simulink model "Battery_Digital_Twin"  (R2026a)
settings: Solver=VariableStepAuto  StopTime=300
undefined symbols (not defined in the file): Battery, BMS, Sensors
libraries: simulink x6
settings Model: Creator=tastytaco  LastModifiedBy=tastytaco

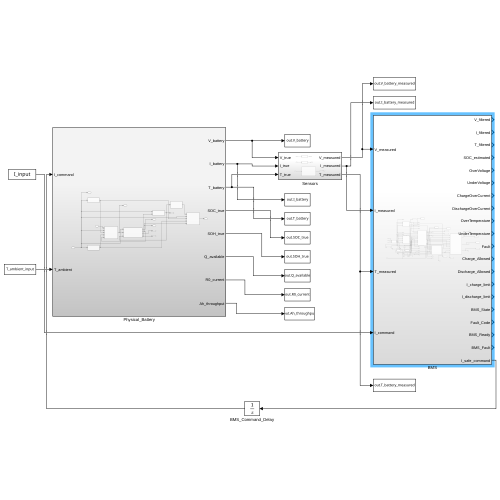
[thumbnail: Simulink's stored preview of the top-level diagram]
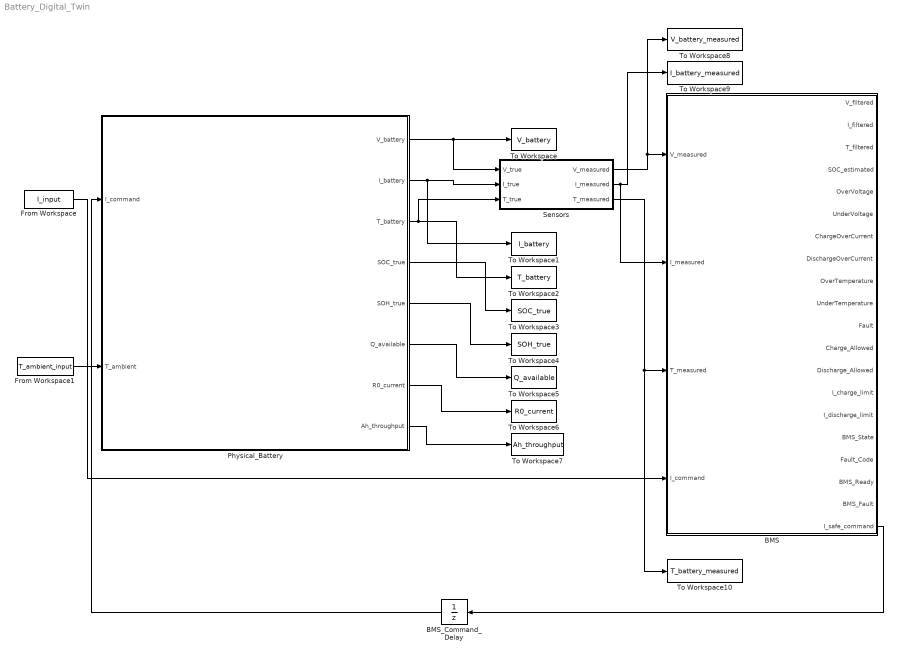
== system Battery_Digital_Twin ==
  BMS : Subsystem
  BMS_Command_Delay : UnitDelay  SampleTime=BMS.Ts
  From Workspace : FromWorkspace  VariableName=I_input
  From Workspace1 : FromWorkspace  VariableName=T_ambient_input
  Physical_Battery : Subsystem
  Sensors : Subsystem
  To Workspace : ToWorkspace  VariableName=V_battery  SaveFormat=Timeseries  SampleTime=-1
  To Workspace1 : ToWorkspace  VariableName=I_battery  SaveFormat=Timeseries  SampleTime=-1
  To Workspace10 : ToWorkspace  VariableName=T_battery_measured  SaveFormat=Timeseries  SampleTime=-1
  To Workspace2 : ToWorkspace  VariableName=T_battery  SaveFormat=Timeseries  SampleTime=-1
  To Workspace3 : ToWorkspace  VariableName=SOC_true  SaveFormat=Timeseries  SampleTime=-1
  To Workspace4 : ToWorkspace  VariableName=SOH_true  SaveFormat=Timeseries  SampleTime=-1
  To Workspace5 : ToWorkspace  VariableName=Q_available  SaveFormat=Timeseries  SampleTime=-1
  To Workspace6 : ToWorkspace  VariableName=R0_current  SaveFormat=Timeseries  SampleTime=-1
  To Workspace7 : ToWorkspace  VariableName=Ah_throughput  SaveFormat=Timeseries  SampleTime=-1
  To Workspace8 : ToWorkspace  VariableName=V_battery_measured  SaveFormat=Timeseries  SampleTime=-1
  To Workspace9 : ToWorkspace  VariableName=I_battery_measured  SaveFormat=Timeseries  SampleTime=-1
  wires:
  Sensors/3(T_measured) -> To Workspace10/1, BMS/3(T_measured)
  Physical_Battery/8(Ah_throughput) -> To Workspace7/1
  Physical_Battery/6(Q_available) -> To Workspace5/1
  Physical_Battery/5(SOH_true) -> To Workspace4/1
  Sensors/1(V_measured) -> BMS/1(V_measured), To Workspace8/1
  Physical_Battery/3(T_battery) -> To Workspace2/1, Sensors/3(T_true)
  Physical_Battery/1(V_battery) -> To Workspace/1, Sensors/1(V_true)
  Physical_Battery/2(I_battery) -> To Workspace1/1, Sensors/2(I_true)
  From Workspace1/1 -> Physical_Battery/2(T_ambient)
  Sensors/2(I_measured) -> BMS/2(I_measured), To Workspace9/1
  Physical_Battery/7(R0_current) -> To Workspace6/1
  Physical_Battery/4(SOC_true) -> To Workspace3/1
  From Workspace/1 -> BMS/4(I_command)
  BMS/20(I_safe_command) -> BMS_Command_Delay/1
  BMS_Command_Delay/1 -> Physical_Battery/1(I_command)

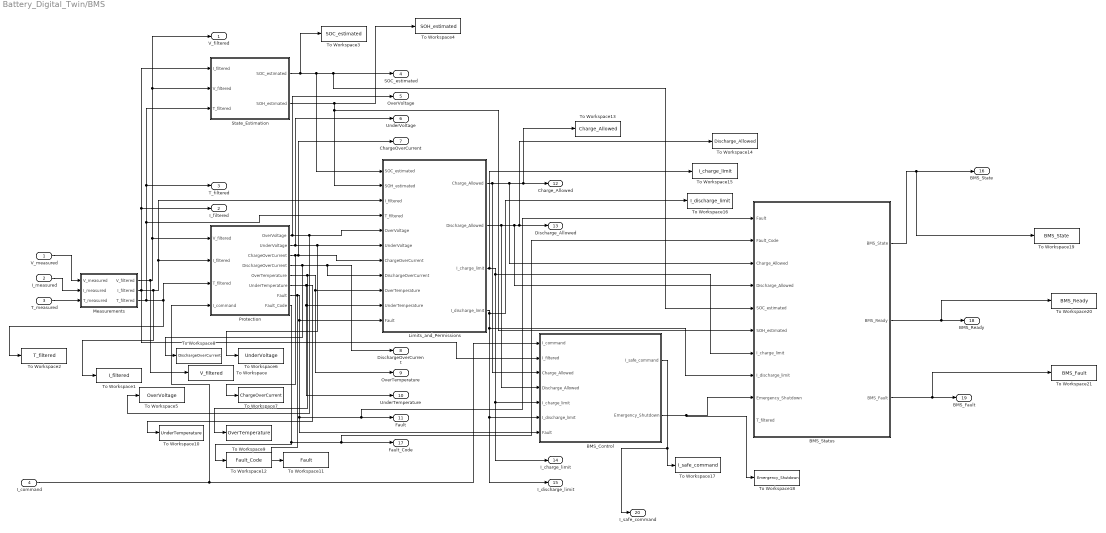
== system Battery_Digital_Twin/BMS ==
  V_measured : Inport
  I_measured : Inport  Port=2
  T_measured : Inport  Port=3
  I_command : Inport  Port=4
  BMS_Control : Subsystem
  BMS_Status : Subsystem
  Limits_and_Permissions : Subsystem
  Measurements : Subsystem
  Protection : Subsystem
  State_Estimation : Subsystem
  To Workspace : ToWorkspace  VariableName=V_filtered  SaveFormat=Timeseries  SampleTime=-1
  To Workspace1 : ToWorkspace  VariableName=I_filtered  SaveFormat=Timeseries  SampleTime=-1
  To Workspace10 : ToWorkspace  VariableName=UnderTemperature  SaveFormat=Timeseries  SampleTime=-1
  To Workspace11 : ToWorkspace  VariableName=Fault  SaveFormat=Timeseries  SampleTime=-1
  To Workspace12 : ToWorkspace  VariableName=Fault_Code  SaveFormat=Timeseries  SampleTime=-1
  To Workspace13 : ToWorkspace  VariableName=Charge_Allowed  SaveFormat=Timeseries  SampleTime=-1
  To Workspace14 : ToWorkspace  VariableName=Discharge_Allowed  SaveFormat=Timeseries  SampleTime=-1
  To Workspace15 : ToWorkspace  VariableName=I_charge_limit  SaveFormat=Timeseries  SampleTime=-1
  To Workspace16 : ToWorkspace  VariableName=I_discharge_limit  SaveFormat=Timeseries  SampleTime=-1
  To Workspace17 : ToWorkspace  VariableName=I_safe_command  SaveFormat=Timeseries  SampleTime=-1
  To Workspace18 : ToWorkspace  VariableName=Emergency_Shutdown  SaveFormat=Timeseries  SampleTime=-1
  To Workspace19 : ToWorkspace  VariableName=BMS_State  SaveFormat=Timeseries  SampleTime=-1
  To Workspace2 : ToWorkspace  VariableName=T_filtered  SaveFormat=Timeseries  SampleTime=-1
  To Workspace20 : ToWorkspace  VariableName=BMS_Ready  SaveFormat=Timeseries  SampleTime=-1
  To Workspace21 : ToWorkspace  VariableName=BMS_Fault  SaveFormat=Timeseries  SampleTime=-1
  To Workspace3 : ToWorkspace  VariableName=SOC_estimated  SaveFormat=Timeseries  SampleTime=-1
  To Workspace4 : ToWorkspace  VariableName=SOH_estimated  SaveFormat=Timeseries  SampleTime=-1
  To Workspace5 : ToWorkspace  VariableName=OverVoltage  SaveFormat=Timeseries  SampleTime=-1
  To Workspace6 : ToWorkspace  VariableName=UnderVoltage  SaveFormat=Timeseries  SampleTime=-1
  To Workspace7 : ToWorkspace  VariableName=ChargeOverCurrent  SaveFormat=Timeseries  SampleTime=-1
  To Workspace8 : ToWorkspace  VariableName=DischargeOverCurrent  SaveFormat=Timeseries  SampleTime=-1
  To Workspace9 : ToWorkspace  VariableName=OverTemperature  SaveFormat=Timeseries  SampleTime=-1
  V_filtered : Outport
  I_filtered : Outport  Port=2
  T_filtered : Outport  Port=3
  SOC_estimated : Outport  Port=4
  OverVoltage : Outport  Port=5
  UnderVoltage : Outport  Port=6
  ChargeOverCurrent : Outport  Port=7
  DischargeOverCurrent : Outport  Port=8
  OverTemperature : Outport  Port=9
  UnderTemperature : Outport  Port=10
  Fault : Outport  Port=11
  Charge_Allowed : Outport  Port=12
  Discharge_Allowed : Outport  Port=13
  I_charge_limit : Outport  Port=14
  I_discharge_limit : Outport  Port=15
  BMS_State : Outport  Port=16
  Fault_Code : Outport  Port=17
  BMS_Ready : Outport  Port=18
  BMS_Fault : Outport  Port=19
  I_safe_command : Outport  Port=20
  wires:
  Limits_and_Permissions/4(I_discharge_limit) -> To Workspace16/1, BMS_Status/8(I_discharge_limit), BMS_Control/6(I_discharge_limit), I_discharge_limit/1
  Limits_and_Permissions/1(Charge_Allowed) -> BMS_Control/3(Charge_Allowed), BMS_Status/3(Charge_Allowed), To Workspace13/1, Charge_Allowed/1
  Protection/8(Fault_Code) -> To Workspace12/1, BMS_Status/2(Fault_Code), Fault_Code/1
  V_measured/1 -> Measurements/1(V_measured)
  T_measured/1 -> Measurements/3(T_measured)
  Limits_and_Permissions/3(I_charge_limit) -> To Workspace15/1, BMS_Status/7(I_charge_limit), BMS_Control/5(I_charge_limit), I_charge_limit/1
  Protection/7(Fault) -> To Workspace11/1, BMS_Status/1(Fault), Fault/1, BMS_Control/7(Fault), Limits_and_Permissions/11(Fault)
  I_measured/1 -> Measurements/2(I_measured)
  Measurements/3(T_filtered) -> State_Estimation/3(T_filtered), T_filtered/1, Limits_and_Permissions/4(T_filtered), To Workspace2/1, Protection/3(T_filtered)
  Measurements/1(V_filtered) -> To Workspace/1, State_Estimation/2(V_filtered), V_filtered/1, Protection/1(V_filtered)
  Measurements/2(I_filtered) -> To Workspace1/1, Protection/2(I_filtered), Limits_and_Permissions/3(I_filtered), State_Estimation/1(I_filtered), I_filtered/1, BMS_Control/2(I_filtered)
  State_Estimation/1(SOC_estimated) -> To Workspace3/1, BMS_Status/5(SOC_estimated), SOC_estimated/1, Limits_and_Permissions/1(SOC_estimated)
  Protection/6(UnderTemperature) -> To Workspace10/1, Limits_and_Permissions/10(UnderTemperature), UnderTemperature/1
  State_Estimation/2(SOH_estimated) -> To Workspace4/1, BMS_Status/6(SOH_estimated), Limits_and_Permissions/2(SOH_estimated)
  Protection/1(OverVoltage) -> OverVoltage/1, To Workspace5/1, Limits_and_Permissions/5(OverVoltage)
  Limits_and_Permissions/2(Discharge_Allowed) -> BMS_Control/4(Discharge_Allowed), BMS_Status/4(Discharge_Allowed), To Workspace14/1, Discharge_Allowed/1
  Protection/5(OverTemperature) -> To Workspace9/1, Limits_and_Permissions/9(OverTemperature), OverTemperature/1
  Protection/2(UnderVoltage) -> UnderVoltage/1, To Workspace6/1, Limits_and_Permissions/6(UnderVoltage)
  Protection/3(ChargeOverCurrent) -> Limits_and_Permissions/7(ChargeOverCurrent), ChargeOverCurrent/1, To Workspace7/1
  Protection/4(DischargeOverCurrent) -> To Workspace8/1, Limits_and_Permissions/8(DischargeOverCurrent), DischargeOverCurrent/1
  BMS_Control/2(Emergency_Shutdown) -> To Workspace18/1, BMS_Status/9(Emergency_Shutdown)
  BMS_Status/1(BMS_State) -> To Workspace19/1, BMS_State/1
  BMS_Status/2(BMS_Ready) -> To Workspace20/1, BMS_Ready/1
  BMS_Status/3(BMS_Fault) -> To Workspace21/1, BMS_Fault/1
  BMS_Control/1(I_safe_command) -> I_safe_command/1, To Workspace17/1
  I_command/1 -> Protection/4(I_command), BMS_Control/1(I_command)

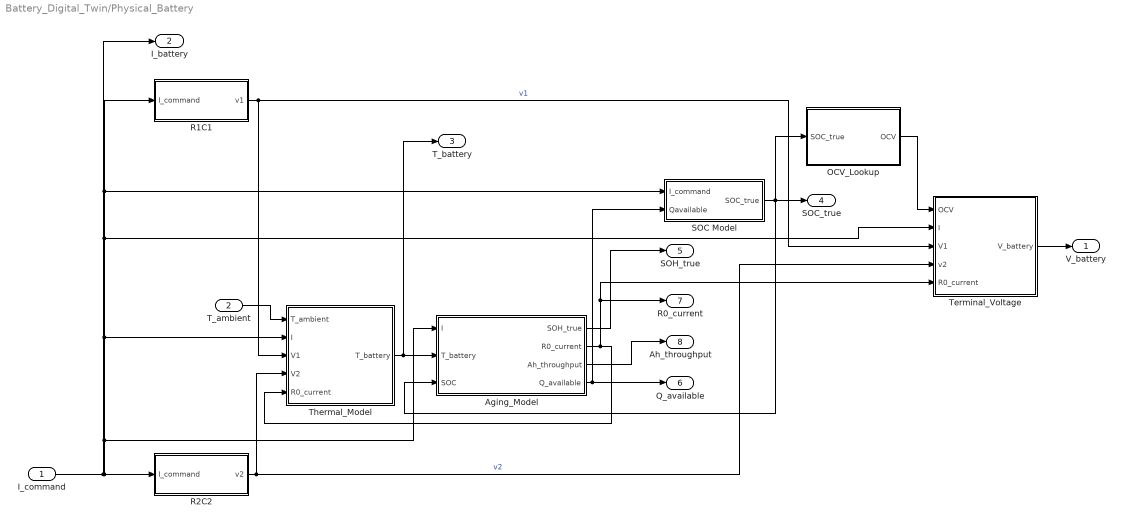
== system Battery_Digital_Twin/Physical_Battery ==
  I_command : Inport
  T_ambient : Inport  Port=2
  " SOC Model" : Subsystem  TreatAsAtomicUnit=on
  Aging_Model : Subsystem
  OCV_Lookup : Subsystem  TreatAsAtomicUnit=on
  R1C1 : Subsystem
  R2C2 : Subsystem
  Terminal_Voltage : Subsystem
  Thermal_Model : Subsystem  TreatAsAtomicUnit=on
  V_battery : Outport
  I_battery : Outport  Port=2
  T_battery : Outport  Port=3
  SOC_true : Outport  Port=4
  SOH_true : Outport  Port=5
  Q_available : Outport  Port=6
  R0_current : Outport  Port=7
  Ah_throughput : Outport  Port=8
  wires:
  Terminal_Voltage/1(V_battery) -> V_battery/1
  Aging_Model/4(Q_available) -> Q_available/1, " SOC Model"/2(Qavailable)
  Aging_Model/3(Ah_throughput) -> Ah_throughput/1
  " SOC Model"/1(SOC_true) -> SOC_true/1, OCV_Lookup/1(SOC_true), Aging_Model/3(SOC)
  Thermal_Model/1(T_battery) -> Aging_Model/2(T_battery), T_battery/1
  R2C2/1(v2) -> Thermal_Model/4(V2), Terminal_Voltage/4(v2)  "v2"
  OCV_Lookup/1(OCV) -> Terminal_Voltage/1(OCV)
  Aging_Model/2(R0_current) -> R0_current/1, Terminal_Voltage/5(R0_current), Thermal_Model/5(R0_current)
  Aging_Model/1(SOH_true) -> SOH_true/1
  T_ambient/1 -> Thermal_Model/1(T_ambient)
  R1C1/1(v1) -> Thermal_Model/3(V1), Terminal_Voltage/3(V1)  "v1"
  I_command/1 -> R1C1/1(I_command), " SOC Model"/1(I_command), Terminal_Voltage/2(I), Thermal_Model/2(I), Aging_Model/1(I), R2C2/1(I_command), I_battery/1

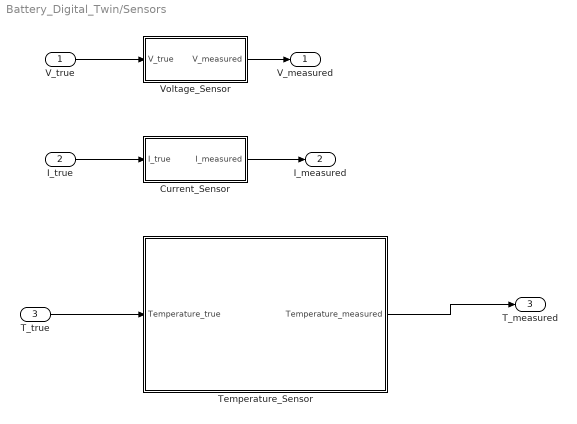
== system Battery_Digital_Twin/Sensors ==
  V_true : Inport
  I_true : Inport  Port=2
  T_true : Inport  Port=3
  Current_Sensor : Subsystem
  Temperature_Sensor : Subsystem
  Voltage_Sensor : Subsystem
  V_measured : Outport
  I_measured : Outport  Port=2
  T_measured : Outport  Port=3
  wires:
  Voltage_Sensor/1(V_measured) -> V_measured/1
  V_true/1 -> Voltage_Sensor/1(V_true)
  Current_Sensor/1(I_measured) -> I_measured/1
  I_true/1 -> Current_Sensor/1(I_true)
  Temperature_Sensor/1(Temperature_measured) -> T_measured/1
  T_true/1 -> Temperature_Sensor/1(Temperature_true)

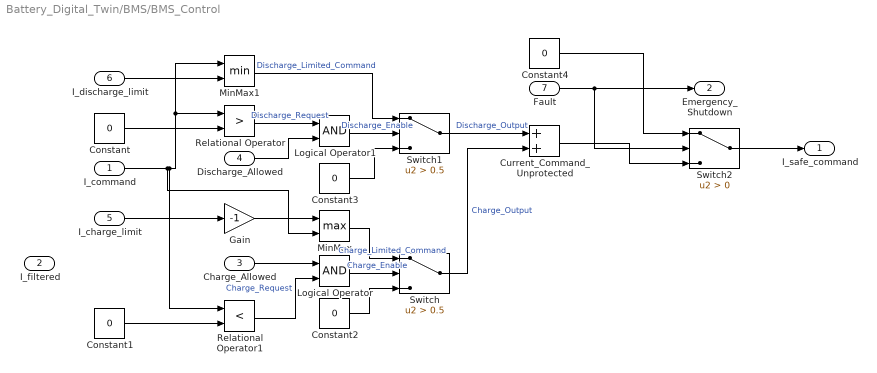
== system Battery_Digital_Twin/BMS/BMS_Control ==
  I_command : Inport
  I_filtered : Inport  Port=2
  Charge_Allowed : Inport  Port=3
  Discharge_Allowed : Inport  Port=4
  I_charge_limit : Inport  Port=5
  I_discharge_limit : Inport  Port=6
  Fault : Inport  Port=7
  Constant{,1..4} (5 alike) : Constant  Value=0
  Current_Command_Unprotected : Sum
  Gain : Gain  Gain=-1
  Logical Operator : Logic  AllPortsSameDT=off  OutDataTypeStr=boolean
  Logical Operator1 : Logic  AllPortsSameDT=off  OutDataTypeStr=boolean
  MinMax : MinMax  Function=max  Inputs=2
  MinMax1 : MinMax  Inputs=2
  Relational Operator : RelationalOperator  Operator=>  OutDataTypeStr=boolean  RndMeth=Simplest  InputSameDT=off
  Relational Operator1 : RelationalOperator  Operator=<  OutDataTypeStr=boolean  RndMeth=Simplest  InputSameDT=off
  Switch : Switch  Criteria=u2 > Threshold  Threshold=0.5  SaturateOnIntegerOverflow=off  InputSameDT=off
  Switch1 : Switch  Criteria=u2 > Threshold  Threshold=0.5  SaturateOnIntegerOverflow=off  InputSameDT=off
  Switch2 : Switch  Criteria=u2 > Threshold  SaturateOnIntegerOverflow=off  InputSameDT=off
  I_safe_command : Outport
  Emergency_Shutdown : Outport  Port=2
  wires:
  Current_Command_Unprotected/1 -> Switch2/3
  Switch/1 -> Current_Command_Unprotected/2  "Charge_Output"
  Switch2/1 -> I_safe_command/1
  Fault/1 -> Emergency_Shutdown/1, Switch2/2
  Switch1/1 -> Current_Command_Unprotected/1  "Discharge_Output"
  Constant2/1 -> Switch/3
  Logical Operator/1 -> Switch/2  "Charge_Enable"
  I_discharge_limit/1 -> MinMax1/2
  MinMax/1 -> Switch/1  "Charge_Limited_Command"
  Constant/1 -> Relational Operator/2
  Charge_Allowed/1 -> Logical Operator/1
  I_charge_limit/1 -> Gain/1
  MinMax1/1 -> Switch1/1  "Discharge_Limited_Command"
  Relational Operator/1 -> Logical Operator1/1  "Discharge_Request"
  Discharge_Allowed/1 -> Logical Operator1/2
  Constant3/1 -> Switch1/3
  I_command/1 -> MinMax1/1, Relational Operator/1, Relational Operator1/1, MinMax/2
  Gain/1 -> MinMax/1
  Constant4/1 -> Switch2/1
  Relational Operator1/1 -> Logical Operator/2  "Charge_Request"
  Constant1/1 -> Relational Operator1/2
  Logical Operator1/1 -> Switch1/2  "Discharge_Enable"

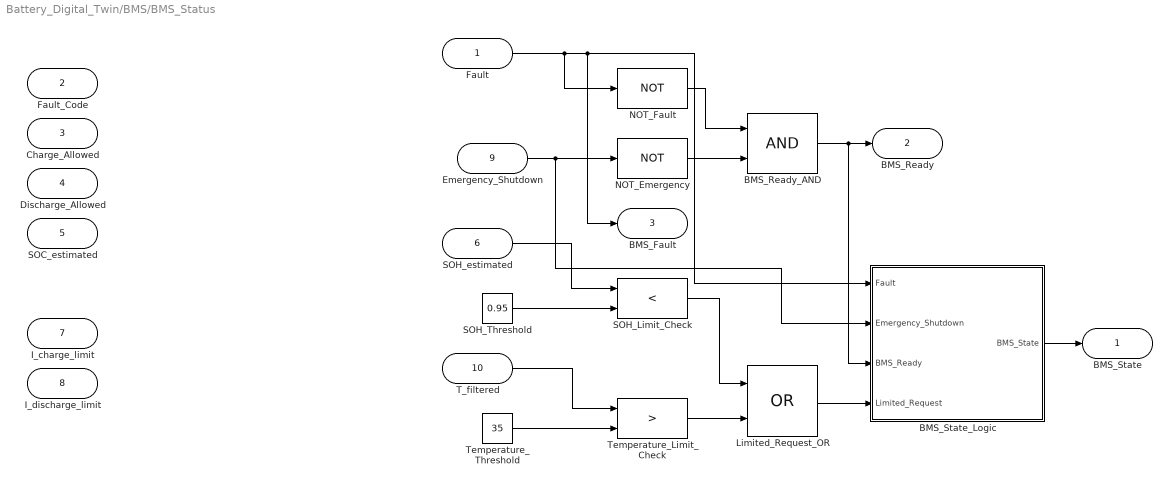
== system Battery_Digital_Twin/BMS/BMS_Status ==
  Fault : Inport
  Fault_Code : Inport  Port=2
  Charge_Allowed : Inport  Port=3
  Discharge_Allowed : Inport  Port=4
  SOC_estimated : Inport  Port=5
  SOH_estimated : Inport  Port=6
  I_charge_limit : Inport  Port=7
  I_discharge_limit : Inport  Port=8
  Emergency_Shutdown : Inport  Port=9
  T_filtered : Inport  Port=10
  BMS_Ready_AND : Logic  AllPortsSameDT=off  OutDataTypeStr=boolean
  BMS_State_Logic : MATLAB Function  TreatAsAtomicUnit=on
  Limited_Request_OR : Logic  Operator=OR  AllPortsSameDT=off  OutDataTypeStr=boolean
  NOT_Emergency : Logic  Operator=NOT  AllPortsSameDT=off  OutDataTypeStr=boolean
  NOT_Fault : Logic  Operator=NOT  AllPortsSameDT=off  OutDataTypeStr=boolean
  SOH_Limit_Check : RelationalOperator  Operator=<  OutDataTypeStr=boolean  RndMeth=Simplest  InputSameDT=off
  SOH_Threshold : Constant  Value=0.95
  Temperature_Limit_Check : RelationalOperator  Operator=>  OutDataTypeStr=boolean  RndMeth=Simplest  InputSameDT=off
  Temperature_Threshold : Constant  Value=35
  BMS_State : Outport
  BMS_Ready : Outport  Port=2
  BMS_Fault : Outport  Port=3
  wires:
  BMS_State_Logic/1(BMS_State) -> BMS_State/1
  Limited_Request_OR/1 -> BMS_State_Logic/4(Limited_Request)
  Temperature_Limit_Check/1 -> Limited_Request_OR/2
  SOH_Limit_Check/1 -> Limited_Request_OR/1
  NOT_Emergency/1 -> BMS_Ready_AND/2
  T_filtered/1 -> Temperature_Limit_Check/1
  SOH_Threshold/1 -> SOH_Limit_Check/2
  SOH_estimated/1 -> SOH_Limit_Check/1
  BMS_Ready_AND/1 -> BMS_Ready/1, BMS_State_Logic/3(BMS_Ready)
  NOT_Fault/1 -> BMS_Ready_AND/1
  Temperature_Threshold/1 -> Temperature_Limit_Check/2
  Emergency_Shutdown/1 -> NOT_Emergency/1, BMS_State_Logic/2(Emergency_Shutdown)
  Fault/1 -> BMS_Fault/1, BMS_State_Logic/1(Fault), NOT_Fault/1

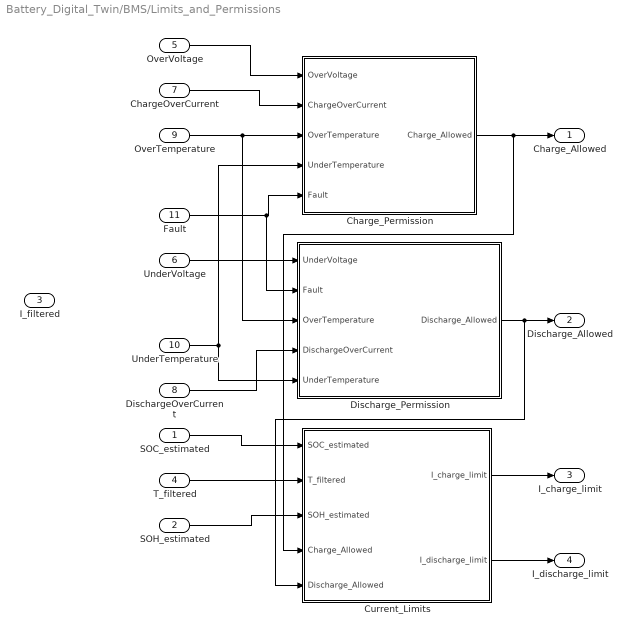
== system Battery_Digital_Twin/BMS/Limits_and_Permissions ==
  SOC_estimated : Inport
  SOH_estimated : Inport  Port=2
  I_filtered : Inport  Port=3
  T_filtered : Inport  Port=4
  OverVoltage : Inport  Port=5
  UnderVoltage : Inport  Port=6
  ChargeOverCurrent : Inport  Port=7
  DischargeOverCurrent : Inport  Port=8
  OverTemperature : Inport  Port=9
  UnderTemperature : Inport  Port=10
  Fault : Inport  Port=11
  Charge_Permission : Subsystem
  Current_Limits : Subsystem
  Discharge_Permission : Subsystem
  Charge_Allowed : Outport
  Discharge_Allowed : Outport  Port=2
  I_charge_limit : Outport  Port=3
  I_discharge_limit : Outport  Port=4
  wires:
  OverVoltage/1 -> Charge_Permission/1(OverVoltage)
  OverTemperature/1 -> Discharge_Permission/3(OverTemperature), Charge_Permission/3(OverTemperature)
  Fault/1 -> Charge_Permission/5(Fault), Discharge_Permission/2(Fault)
  Current_Limits/2(I_discharge_limit) -> I_discharge_limit/1
  UnderTemperature/1 -> Charge_Permission/4(UnderTemperature), Discharge_Permission/5(UnderTemperature)
  Discharge_Permission/1(Discharge_Allowed) -> Current_Limits/5(Discharge_Allowed), Discharge_Allowed/1
  DischargeOverCurrent/1 -> Discharge_Permission/4(DischargeOverCurrent)
  SOC_estimated/1 -> Current_Limits/1(SOC_estimated)
  ChargeOverCurrent/1 -> Charge_Permission/2(ChargeOverCurrent)
  UnderVoltage/1 -> Discharge_Permission/1(UnderVoltage)
  Current_Limits/1(I_charge_limit) -> I_charge_limit/1
  Charge_Permission/1(Charge_Allowed) -> Current_Limits/4(Charge_Allowed), Charge_Allowed/1
  T_filtered/1 -> Current_Limits/2(T_filtered)
  SOH_estimated/1 -> Current_Limits/3(SOH_estimated)

== system Battery_Digital_Twin/BMS/Measurements ==
  V_measured : Inport
  I_measured : Inport  Port=2
  T_measured : Inport  Port=3
  Current_Filter : Subsystem
  Temperature_Filter : Subsystem
  Voltage_Filter : Subsystem
  V_filtered : Outport
  I_filtered : Outport  Port=2
  T_filtered : Outport  Port=3
  wires:
  Temperature_Filter/1(V_filtered) -> T_filtered/1
  Voltage_Filter/1(V_filtered) -> V_filtered/1
  Current_Filter/1(V_filtered) -> I_filtered/1
  I_measured/1 -> Current_Filter/1(V_measured)
  T_measured/1 -> Temperature_Filter/1(V_measured)
  V_measured/1 -> Voltage_Filter/1(V_measured)

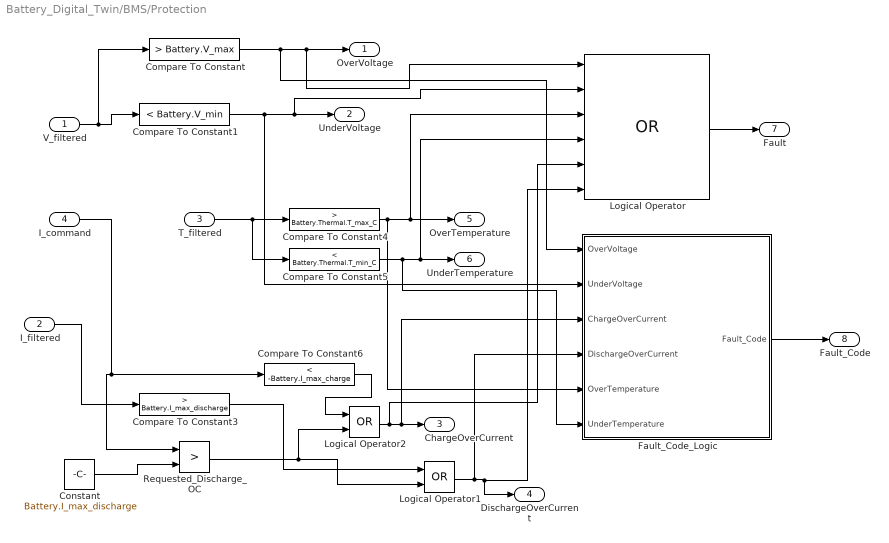
== system Battery_Digital_Twin/BMS/Protection ==
  V_filtered : Inport
  I_filtered : Inport  Port=2
  T_filtered : Inport  Port=3
  I_command : Inport  Port=4
  Compare To Constant : simulink/Logic and Bit Operations/Compare To Constant  relop=>  const=Battery.V_max  OutDataTypeStr=boolean
  Compare To Constant1 : simulink/Logic and Bit Operations/Compare To Constant  relop=<  const=Battery.V_min  OutDataTypeStr=boolean
  Compare To Constant3 : simulink/Logic and Bit Operations/Compare To Constant  relop=>  const=Battery.I_max_discharge  OutDataTypeStr=boolean
  Compare To Constant4 : simulink/Logic and Bit Operations/Compare To Constant  relop=>  const=Battery.Thermal.T_max_C  OutDataTypeStr=boolean
  Compare To Constant5 : simulink/Logic and Bit Operations/Compare To Constant  relop=<  const=Battery.Thermal.T_min_C  OutDataTypeStr=boolean
  Compare To Constant6 : simulink/Logic and Bit Operations/Compare To Constant  relop=<  const=-Battery.I_max_charge  OutDataTypeStr=boolean
  Constant : Constant  Value=Battery.I_max_discharge
  Fault_Code_Logic : Subsystem
  Logical Operator : Logic  Operator=OR  Inputs=6  AllPortsSameDT=off  OutDataTypeStr=boolean
  Logical Operator1 : Logic  Operator=OR  AllPortsSameDT=off  OutDataTypeStr=boolean
  Logical Operator2 : Logic  Operator=OR  AllPortsSameDT=off  OutDataTypeStr=boolean
  Requested_Discharge_OC : RelationalOperator  Operator=>  OutDataTypeStr=boolean  RndMeth=Simplest  InputSameDT=off
  OverVoltage : Outport
  UnderVoltage : Outport  Port=2
  ChargeOverCurrent : Outport  Port=3
  DischargeOverCurrent : Outport  Port=4
  OverTemperature : Outport  Port=5
  UnderTemperature : Outport  Port=6
  Fault : Outport  Port=7
  Fault_Code : Outport  Port=8
  wires:
  V_filtered/1 -> Compare To Constant1/1, Compare To Constant/1
  Compare To Constant1/1 -> Fault_Code_Logic/2(UnderVoltage), Logical Operator/2, UnderVoltage/1
  Compare To Constant/1 -> Fault_Code_Logic/1(OverVoltage), Logical Operator/1, OverVoltage/1
  I_filtered/1 -> Compare To Constant3/1
  Compare To Constant3/1 -> Logical Operator1/1
  T_filtered/1 -> Compare To Constant5/1, Compare To Constant4/1
  Compare To Constant4/1 -> Logical Operator/3, OverTemperature/1, Fault_Code_Logic/5(OverTemperature)
  Compare To Constant5/1 -> Fault_Code_Logic/6(UnderTemperature), Logical Operator/4, UnderTemperature/1
  Logical Operator/1 -> Fault/1
  Fault_Code_Logic/1(Fault_Code) -> Fault_Code/1
  Constant/1 -> Requested_Discharge_OC/2
  I_command/1 -> Requested_Discharge_OC/1, Compare To Constant6/1
  Requested_Discharge_OC/1 -> Logical Operator2/2, Logical Operator1/2
  Logical Operator1/1 -> Fault_Code_Logic/4(DischargeOverCurrent), Logical Operator/6, DischargeOverCurrent/1
  Compare To Constant6/1 -> Logical Operator2/1
  Logical Operator2/1 -> Logical Operator/5, Fault_Code_Logic/3(ChargeOverCurrent), ChargeOverCurrent/1

== system Battery_Digital_Twin/BMS/State_Estimation ==
  I_filtered : Inport
  V_filtered : Inport  Port=2
  T_filtered : Inport  Port=3
  SOC_Estimator : Subsystem
  SOH_Estimator : Subsystem
  SOC_estimated : Outport
  SOH_estimated : Outport  Port=2
  wires:
  I_filtered/1 -> SOH_Estimator/2(I_filtered), SOC_Estimator/1(I_filtered)
  SOC_Estimator/1(SOC_estimated) -> SOC_estimated/1
  V_filtered/1 -> SOH_Estimator/1(V_filtered)
  T_filtered/1 -> SOH_Estimator/3(T_filtered)
  SOH_Estimator/1(SOH_estimated) -> SOH_estimated/1

== system Battery_Digital_Twin/Physical_Battery/ SOC Model ==
  I_command : Inport
  Qavailable : Inport  Port=2
  Divide : Product  Inputs=*/
  Gain1 : Gain  Gain=-1/3600
  IC : Integrator  InitialCondition=Battery.SOC_initial
  Q_available : Gain  Gain=Battery.eta_discharge
  Saturation : Saturate  UpperLimit=1  LowerLimit=0
  SOC_true : Outport
  wires:
  Saturation/1 -> SOC_true/1
  IC/1 -> Saturation/1
  Q_available/1 -> Divide/1
  Qavailable/1 -> Divide/2
  I_command/1 -> Q_available/1
  Gain1/1 -> IC/1
  Divide/1 -> Gain1/1

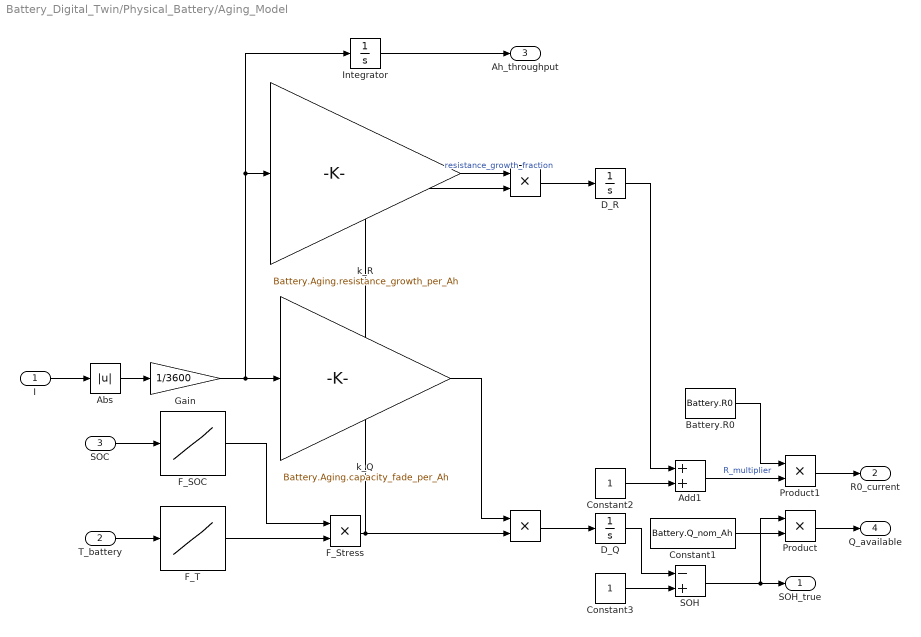
== system Battery_Digital_Twin/Physical_Battery/Aging_Model ==
  I : Inport
  T_battery : Inport  Port=2
  SOC : Inport  Port=3
  " " : Product
  "  " : Product
  Abs : Abs  SaturateOnIntegerOverflow=off
  Add1 : Sum
  "Battery.R0 " : Constant  Value=Battery.R0
  Constant1 : Constant  Value=Battery.Q_nom_Ah
  Constant2 : Constant
  Constant3 : Constant
  D_Q : Integrator
  D_R : Integrator
  F_SOC : Lookup_n-D  NumberOfTableDimensions=1  BreakpointsForDimension1=[0 0.1 0.2 0.4 0.6 0.8 0.9 1.0]  Table=[1.5 1.2 1.05 1.0 1.0 1.05 1.2 1.5]  InternalRulePriority=Speed  RndMeth=Simplest
  F_Stress : Product
  "F_T " : Lookup_n-D  NumberOfTableDimensions=1  BreakpointsForDimension1=[0 10 20 25 30 35 40 45]  Table=[1.5 1.2 1.05 1.0 1.05 1.2 1.5 2.0]  InternalRulePriority=Speed  RndMeth=Simplest
  Gain : Gain  Gain=1/3600
  Integrator : Integrator
  Product : Product
  Product1 : Product
  SOH : Sum  Inputs=-+
  k_Q : Gain  Gain=Battery.Aging.capacity_fade_per_Ah
  k_R : Gain  Gain=Battery.Aging.resistance_growth_per_Ah
  SOH_true : Outport
  R0_current : Outport  Port=2
  Ah_throughput : Outport  Port=3
  Q_available : Outport  Port=4
  wires:
  Product/1 -> Q_available/1
  Product1/1 -> R0_current/1
  Add1/1 -> Product1/2  "R_multiplier"
  Constant3/1 -> SOH/2
  D_Q/1 -> SOH/1
  D_R/1 -> Add1/1
  I/1 -> Abs/1
  F_Stress/1 -> "  "/2, " "/2
  SOH/1 -> SOH_true/1, Product/1
  Constant1/1 -> Product/2
  SOC/1 -> F_SOC/1
  "Battery.R0 "/1 -> Product1/1
  T_battery/1 -> "F_T "/1
  k_R/1 -> "  "/1  "resistance_growth_fraction"
  Gain/1 -> k_R/1, Integrator/1, k_Q/1
  "  "/1 -> D_R/1
  "F_T "/1 -> F_Stress/2
  Abs/1 -> Gain/1
  Integrator/1 -> Ah_throughput/1
  Constant2/1 -> Add1/2
  k_Q/1 -> " "/1
  F_SOC/1 -> F_Stress/1
  " "/1 -> D_Q/1

== system Battery_Digital_Twin/Physical_Battery/OCV_Lookup ==
  SOC_true : Inport
  1-D Lookup Table : Lookup_n-D  NumberOfTableDimensions=1  BreakpointsForDimension1=Battery.OCV.SOC  Table=Battery.OCV.Voltage  InternalRulePriority=Speed  RndMeth=Simplest
  OCV : Outport
  wires:
  SOC_true/1 -> 1-D Lookup Table/1
  1-D Lookup Table/1 -> OCV/1

== system Battery_Digital_Twin/Physical_Battery/R1C1 ==
  I_command : Inport
  Add : Sum  Inputs=+-
  Gain : Gain  Gain=1/(Battery.R1*Battery.C1)
  Gain1 : Gain  Gain=1/Battery.C1
  Integrator : Integrator
  v1 : Outport
  wires:
  I_command/1 -> Gain1/1
  Gain1/1 -> Add/1
  Gain/1 -> Add/2
  Add/1 -> Integrator/1
  Integrator/1 -> Gain/1, v1/1

== system Battery_Digital_Twin/Physical_Battery/R2C2 ==
  I_command : Inport
  Add : Sum  Inputs=+-
  Gain : Gain  Gain=1/(Battery.R2*Battery.C2)
  Gain1 : Gain  Gain=1/Battery.C2
  Integrator : Integrator
  v2 : Outport
  wires:
  I_command/1 -> Gain1/1
  Gain1/1 -> Add/1
  Gain/1 -> Add/2
  Add/1 -> Integrator/1
  Integrator/1 -> Gain/1, v2/1

== system Battery_Digital_Twin/Physical_Battery/Terminal_Voltage ==
  OCV : Inport
  I : Inport  Port=2
  V1 : Inport  Port=3
  v2 : Inport  Port=4
  R0_current : Inport  Port=5
  Add : Sum  Inputs=+---
  Product : Product
  V_battery : Outport
  wires:
  v2/1 -> Add/4
  Add/1 -> V_battery/1
  V1/1 -> Add/3
  Product/1 -> Add/2
  R0_current/1 -> Product/2
  OCV/1 -> Add/1
  I/1 -> Product/1

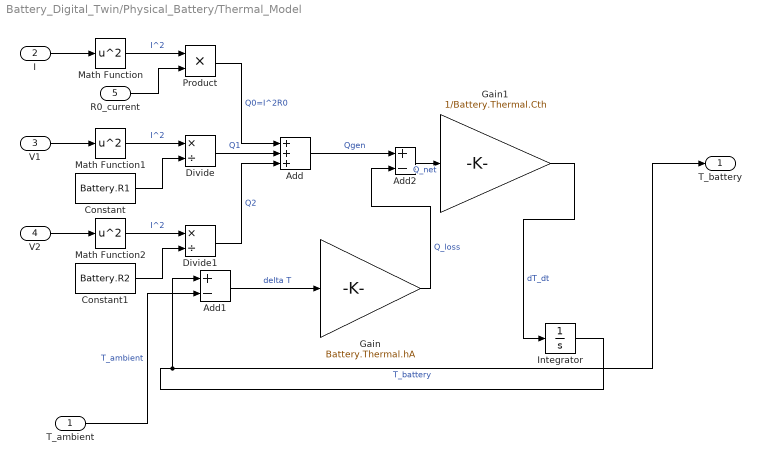
== system Battery_Digital_Twin/Physical_Battery/Thermal_Model ==
  T_ambient : Inport
  I : Inport  Port=2
  V1 : Inport  Port=3
  V2 : Inport  Port=4
  R0_current : Inport  Port=5
  Add : Sum  Inputs=+++
  Add1 : Sum  Inputs=+-
  Add2 : Sum  Inputs=+-
  Constant : Constant  Value=Battery.R1
  Constant1 : Constant  Value=Battery.R2
  Divide : Product  Inputs=*/
  Divide1 : Product  Inputs=*/
  Gain : Gain  Gain=Battery.Thermal.hA
  Gain1 : Gain  Gain=1/Battery.Thermal.Cth
  Integrator : Integrator  InitialCondition=Battery.T_initial_C
  Math Function : Math  Operator=square
  Math Function1 : Math  Operator=square
  Math Function2 : Math  Operator=square
  Product : Product
  T_battery : Outport
  wires:
  Add2/1 -> Gain1/1  "Q_net"
  Gain1/1 -> Integrator/1  "dT_dt"
  Gain/1 -> Add2/2  "Q_loss"
  Add/1 -> Add2/1  "Qgen"
  Add1/1 -> Gain/1  "delta T"
  I/1 -> Math Function/1
  V2/1 -> Math Function2/1
  V1/1 -> Math Function1/1
  Divide1/1 -> Add/3  "Q2"
  Math Function/1 -> Product/1  "I^2"
  Divide/1 -> Add/2  "Q1"
  R0_current/1 -> Product/2
  Constant/1 -> Divide/2
  Math Function2/1 -> Divide1/1  "I^2"
  Math Function1/1 -> Divide/1  "I^2"
  Constant1/1 -> Divide1/2
  T_ambient/1 -> Add1/2  "T_ambient"
  Integrator/1 -> T_battery/1, Add1/1  "T_battery"
  Product/1 -> Add/1  "Q0=I^2R0"

== system Battery_Digital_Twin/Sensors/Current_Sensor ==
  I_true : Inport
  Add : Sum  Inputs=+++
  Current_Bias : Constant  Value=Sensors.Current.Bias_A
  Current_Noise : RandomNumber  Mean=Sensors.Current.Noise_Mean_A  Variance=Sensors.Current.Noise_Variance_A2  Seed=12345  SampleTime=Sensors.Current.SampleTime
  I_measured : Outport
  wires:
  Current_Bias/1 -> Add/1
  Current_Noise/1 -> Add/3
  Add/1 -> I_measured/1
  I_true/1 -> Add/2

== system Battery_Digital_Twin/Sensors/Temperature_Sensor ==
  Temperature_true : Inport
  Add : Sum  Inputs=+++
  Temperature_Bias : Constant  Value=Sensors.Temperature.Bias_C
  Temperature_Noise : RandomNumber  Mean=Sensors.Temperature.Noise_Mean_C  Variance=Sensors.Temperature.Noise_Variance_C2  Seed=12345  SampleTime=Sensors.Temperature.SampleTime
  Temperature_measured : Outport
  wires:
  Temperature_true/1 -> Add/2
  Add/1 -> Temperature_measured/1
  Temperature_Noise/1 -> Add/3
  Temperature_Bias/1 -> Add/1

== system Battery_Digital_Twin/Sensors/Voltage_Sensor ==
  V_true : Inport
  Add : Sum  Inputs=+++
  Voltage_Bias : Constant  Value=Sensors.Voltage.Bias_V
  Voltage_Noise : RandomNumber  Mean=Sensors.Voltage.Noise_Mean_V  Variance=Sensors.Voltage.Noise_Variance_V2  Seed=12345  SampleTime=Sensors.Voltage.SampleTime
  V_measured : Outport
  wires:
  V_true/1 -> Add/2
  Add/1 -> V_measured/1
  Voltage_Noise/1 -> Add/3
  Voltage_Bias/1 -> Add/1

== system Battery_Digital_Twin/BMS/Limits_and_Permissions/Charge_Permission ==
  OverVoltage : Inport
  ChargeOverCurrent : Inport  Port=2
  OverTemperature : Inport  Port=3
  UnderTemperature : Inport  Port=4
  Fault : Inport  Port=5
  Logical Operator : Logic  Operator=OR  Inputs=5  AllPortsSameDT=off  OutDataTypeStr=boolean
  Logical Operator1 : Logic  Operator=NOT  AllPortsSameDT=off  OutDataTypeStr=boolean
  Charge_Allowed : Outport
  wires:
  Fault/1 -> Logical Operator/5
  UnderTemperature/1 -> Logical Operator/4
  Logical Operator1/1 -> Charge_Allowed/1
  Logical Operator/1 -> Logical Operator1/1
  OverTemperature/1 -> Logical Operator/3
  ChargeOverCurrent/1 -> Logical Operator/2
  OverVoltage/1 -> Logical Operator/1

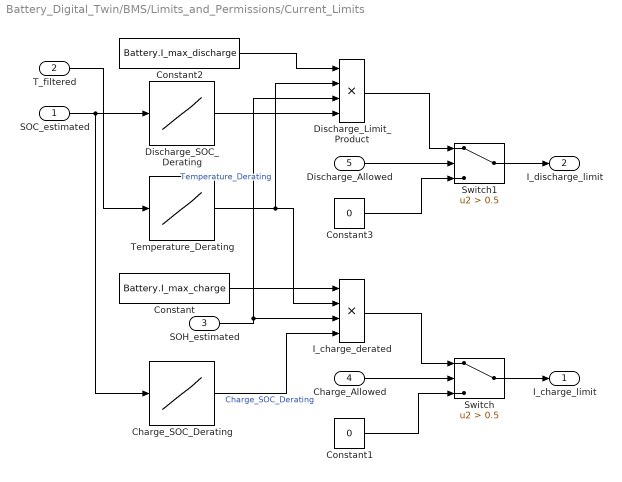
== system Battery_Digital_Twin/BMS/Limits_and_Permissions/Current_Limits ==
  SOC_estimated : Inport
  T_filtered : Inport  Port=2
  SOH_estimated : Inport  Port=3
  Charge_Allowed : Inport  Port=4
  Discharge_Allowed : Inport  Port=5
  Charge_SOC_Derating : Lookup_n-D  NumberOfTableDimensions=1  BreakpointsForDimension1=[0 0.10 0.20 0.50 0.80 0.90 0.95 0.98 1.00]  Table=[1.0 1.0 1.0 1.0 1.0 0.8 0.5 0.2 0.0]  InternalRulePriority=Speed  RndMeth=Simplest
  Constant : Constant  Value=Battery.I_max_charge
  Constant1 : Constant  Value=0
  Constant2 : Constant  Value=Battery.I_max_discharge
  Constant3 : Constant  Value=0
  Discharge_Limit_Product : Product  Inputs=4
  Discharge_SOC_Derating : Lookup_n-D  NumberOfTableDimensions=1  BreakpointsForDimension1=[0 0.02 0.05 0.10 0.20 0.50 0.80 1.00]  Table=[0.0 0.2 0.5 0.8 1.0 1.0 1.0 1.0]  InternalRulePriority=Speed  RndMeth=Simplest
  I_charge_derated : Product  Inputs=4
  Switch : Switch  Criteria=u2 > Threshold  Threshold=0.5  SaturateOnIntegerOverflow=off  InputSameDT=off
  Switch1 : Switch  Criteria=u2 > Threshold  Threshold=0.5  SaturateOnIntegerOverflow=off  InputSameDT=off
  Temperature_Derating : Lookup_n-D  NumberOfTableDimensions=1  BreakpointsForDimension1=[0 10 20 25 35 40 45]  Table=[0.5 0.8 1.0 1.0 0.9 0.5 0]  InternalRulePriority=Speed  RndMeth=Simplest
  I_charge_limit : Outport
  I_discharge_limit : Outport  Port=2
  wires:
  Switch/1 -> I_charge_limit/1
  Constant1/1 -> Switch/3
  T_filtered/1 -> Temperature_Derating/1
  Discharge_SOC_Derating/1 -> Discharge_Limit_Product/4
  SOC_estimated/1 -> Discharge_SOC_Derating/1, Charge_SOC_Derating/1
  Switch1/1 -> I_discharge_limit/1
  I_charge_derated/1 -> Switch/1
  Constant2/1 -> Discharge_Limit_Product/1
  Temperature_Derating/1 -> Discharge_Limit_Product/2, I_charge_derated/2  "Temperature_Derating"
  Discharge_Allowed/1 -> Switch1/2
  Constant/1 -> I_charge_derated/1
  SOH_estimated/1 -> Discharge_Limit_Product/3, I_charge_derated/3
  Charge_SOC_Derating/1 -> I_charge_derated/4  "Charge_SOC_Derating"
  Discharge_Limit_Product/1 -> Switch1/1
  Constant3/1 -> Switch1/3
  Charge_Allowed/1 -> Switch/2

== system Battery_Digital_Twin/BMS/Limits_and_Permissions/Discharge_Permission ==
  UnderVoltage : Inport
  Fault : Inport  Port=2
  OverTemperature : Inport  Port=3
  DischargeOverCurrent : Inport  Port=4
  UnderTemperature : Inport  Port=5
  Logical Operator : Logic  Operator=OR  Inputs=5  AllPortsSameDT=off  OutDataTypeStr=boolean
  Logical Operator1 : Logic  Operator=NOT  AllPortsSameDT=off  OutDataTypeStr=boolean
  Discharge_Allowed : Outport
  wires:
  Logical Operator1/1 -> Discharge_Allowed/1
  Logical Operator/1 -> Logical Operator1/1
  UnderTemperature/1 -> Logical Operator/5
  OverTemperature/1 -> Logical Operator/4
  Fault/1 -> Logical Operator/3
  DischargeOverCurrent/1 -> Logical Operator/2
  UnderVoltage/1 -> Logical Operator/1

== system Battery_Digital_Twin/BMS/Measurements/Current_Filter ==
  V_measured : Inport
  Add : Sum
  Gain : Gain  Gain=1 - BMS.Filter.Alpha
  Gain1 : Gain  Gain=BMS.Filter.Alpha
  Unit Delay : UnitDelay  SampleTime=BMS.Ts
  V_filtered : Outport
  wires:
  Add/1 -> V_filtered/1, Unit Delay/1
  Gain/1 -> Add/1
  Unit Delay/1 -> Gain1/1
  Gain1/1 -> Add/2
  V_measured/1 -> Gain/1

== system Battery_Digital_Twin/BMS/Measurements/Temperature_Filter ==
  V_measured : Inport
  Add : Sum
  Gain : Gain  Gain=1 - BMS.Filter.Alpha
  Gain1 : Gain  Gain=BMS.Filter.Alpha
  Unit Delay : UnitDelay  InitialCondition=Battery.T_initial_C  SampleTime=BMS.Ts
  V_filtered : Outport
  wires:
  V_measured/1 -> Gain/1
  Gain1/1 -> Add/2
  Unit Delay/1 -> Gain1/1
  Gain/1 -> Add/1
  Add/1 -> Unit Delay/1, V_filtered/1

== system Battery_Digital_Twin/BMS/Measurements/Voltage_Filter ==
  V_measured : Inport
  Add : Sum
  Gain : Gain  Gain=1 - BMS.Filter.Alpha
  Gain1 : Gain  Gain=BMS.Filter.Alpha
  Unit Delay : UnitDelay  InitialCondition=Battery.V_nom  SampleTime=BMS.Ts
  V_filtered : Outport
  wires:
  Add/1 -> V_filtered/1, Unit Delay/1
  Gain/1 -> Add/1
  Unit Delay/1 -> Gain1/1
  Gain1/1 -> Add/2
  V_measured/1 -> Gain/1

== system Battery_Digital_Twin/BMS/Protection/Fault_Code_Logic ==
  OverVoltage : Inport
  UnderVoltage : Inport  Port=2
  ChargeOverCurrent : Inport  Port=3
  DischargeOverCurrent : Inport  Port=4
  OverTemperature : Inport  Port=5
  UnderTemperature : Inport  Port=6
  MATLAB Function : MATLAB Function  TreatAsAtomicUnit=on
  Fault_Code : Outport
  wires:
  MATLAB Function/1(Fault_Code) -> Fault_Code/1
  OverVoltage/1 -> MATLAB Function/1(OverVoltage)
  UnderVoltage/1 -> MATLAB Function/2(UnderVoltage)
  ChargeOverCurrent/1 -> MATLAB Function/3(ChargeOverCurrent)
  DischargeOverCurrent/1 -> MATLAB Function/4(DischargeOverCurrent)
  OverTemperature/1 -> MATLAB Function/5(OverTemperature)
  UnderTemperature/1 -> MATLAB Function/6(UnderTemperature)

== system Battery_Digital_Twin/BMS/State_Estimation/SOC_Estimator ==
  I_filtered : Inport
  Gain : Gain  Gain=-BMS.SOC.Efficiency/(3600*Battery.Q_nom_Ah)
  Integrator : Integrator  InitialCondition=Battery.SOC_initial
  Saturation : Saturate  UpperLimit=BMS.SOC.Max  LowerLimit=BMS.SOC.Min
  SOC_estimated : Outport
  wires:
  I_filtered/1 -> Gain/1
  Gain/1 -> Integrator/1
  Integrator/1 -> Saturation/1
  Saturation/1 -> SOC_estimated/1

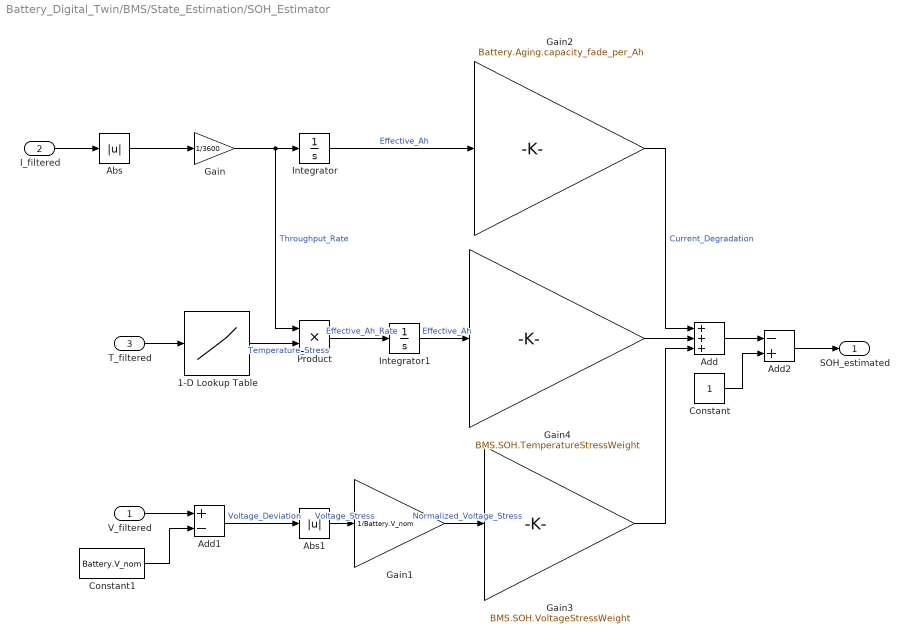
== system Battery_Digital_Twin/BMS/State_Estimation/SOH_Estimator ==
  V_filtered : Inport
  I_filtered : Inport  Port=2
  T_filtered : Inport  Port=3
  1-D Lookup Table : Lookup_n-D  NumberOfTableDimensions=1  BreakpointsForDimension1=[0 10 20 25 30 35 40 45]  Table=[1.5 1.2 1.05 1.0 1.05 1.2 1.5 2.0]  InternalRulePriority=Speed  RndMeth=Simplest
  Abs : Abs  SaturateOnIntegerOverflow=off
  Abs1 : Abs  SaturateOnIntegerOverflow=off
  Add : Sum  Inputs=+++
  Add1 : Sum  Inputs=+-
  Add2 : Sum  Inputs=-+
  Constant : Constant
  Constant1 : Constant  Value=Battery.V_nom
  Gain : Gain  Gain=1/3600
  Gain1 : Gain  Gain=1/Battery.V_nom
  Gain2 : Gain  Gain=Battery.Aging.capacity_fade_per_Ah
  Gain3 : Gain  Gain=BMS.SOH.VoltageStressWeight
  Gain4 : Gain  Gain=BMS.SOH.TemperatureStressWeight
  Integrator : Integrator
  Integrator1 : Integrator
  Product : Product
  SOH_estimated : Outport
  wires:
  Add2/1 -> SOH_estimated/1
  Constant/1 -> Add2/2
  Gain3/1 -> Add/3
  V_filtered/1 -> Add1/1
  Constant1/1 -> Add1/2
  Abs/1 -> Gain/1
  Gain4/1 -> Add/2
  Gain2/1 -> Add/1  "Current_Degradation"
  T_filtered/1 -> 1-D Lookup Table/1
  Gain/1 -> Product/1, Integrator/1  "Throughput_Rate"
  Add1/1 -> Abs1/1  "Voltage_Deviation"
  1-D Lookup Table/1 -> Product/2  "Temperature_Stress"
  Integrator/1 -> Gain2/1  "Effective_Ah"
  Gain1/1 -> Gain3/1  "Normalized_Voltage_Stress"
  Integrator1/1 -> Gain4/1  "Effective_Ah"
  Add/1 -> Add2/1
  Product/1 -> Integrator1/1  "Effective_Ah_Rate"
  I_filtered/1 -> Abs/1
  Abs1/1 -> Gain1/1  "Voltage_Stress"

== matlab function Battery_Digital_Twin/BMS/BMS_Status/BMS_State_Logic ==
  data: Fault input; BMS_State output; Emergency_Shutdown input; BMS_Ready input; Limited_Request input
function BMS_State = fcn(Fault, Emergency_Shutdown, BMS_Ready, Limited_Request)

% BMS State Codes
% 0 = INIT
% 1 = NORMAL
% 2 = LIMITED
% 3 = FAULT
% 4 = SHUTDOWN

% Highest priority: Emergency Shutdown
if Emergency_Shutdown
    BMS_State = 4;

% Protection fault
elseif Fault
    BMS_State = 3;

% BMS not ready
elseif ~BMS_Ready
    BMS_State = 0;

% Battery operating under limitation
elseif Limited_Request
    BMS_State = 2;

% Normal operation
else
    BMS_State = 1;
end

end

== matlab function Battery_Digital_Twin/BMS/Protection/Fault_Code_Logic/MATLAB Function ==
  data: OverVoltage input; Fault_Code output; UnderVoltage input; ChargeOverCurrent input; DischargeOverCurrent input; OverTemperature input; UnderTemperature input
function Fault_Code = fcn( ...
    OverVoltage, ...
    UnderVoltage, ...
    ChargeOverCurrent, ...
    DischargeOverCurrent, ...
    OverTemperature, ...
    UnderTemperature)

% Fault code:
%
% 0 = No fault
% 1 = Over voltage
% 2 = Under voltage
% 3 = Charge over-current
% 4 = Discharge over-current
% 5 = Over temperature
% 6 = Under temperature
% 7 = Multiple faults

faultCount = ...
    OverVoltage + ...
    UnderVoltage + ...
    ChargeOverCurrent + ...
    DischargeOverCurrent + ...
    OverTemperature + ...
    UnderTemperature;

if faultCount == 0

    Fault_Code = 0;

elseif faultCount > 1

    Fault_Code = 7;

elseif OverVoltage

    Fault_Code = 1;

elseif UnderVoltage

    Fault_Code = 2;

elseif ChargeOverCurrent

    Fault_Code = 3;

elseif DischargeOverCurrent

    Fault_Code = 4;

elseif OverTemperature

    Fault_Code = 5;

elseif UnderTemperature

    Fault_Code = 6;

else

    Fault_Code = 0;

end

end
